simulink model "Task1_SARADC"  (R2026a)
settings: Solver=ode45  StopTime=2000.0000e-009  RelTol=1e-1
values from neighbouring files (symbols this model uses):
  clkper = 10e-9    (= 1e-08)    [Task1_SAR_ADC.m]
  nbit = 8    [Task1_SAR_ADC.m]
undefined symbols (not defined in the file or in its folder): coeff, ramp_slope
libraries: simulink_extras x18, simulink x1
settings Model: Creator=DELL  LastModifiedBy=DELL

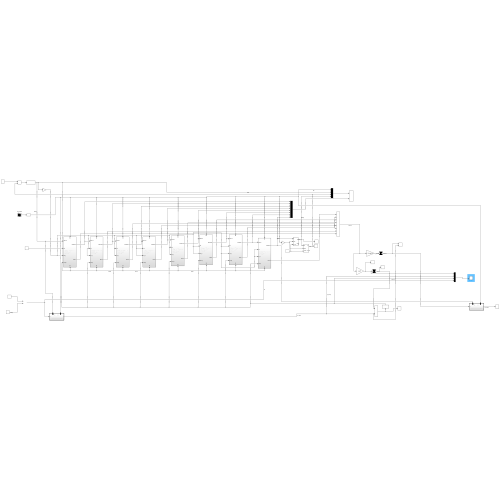
[thumbnail: Simulink's stored preview of the top-level diagram]
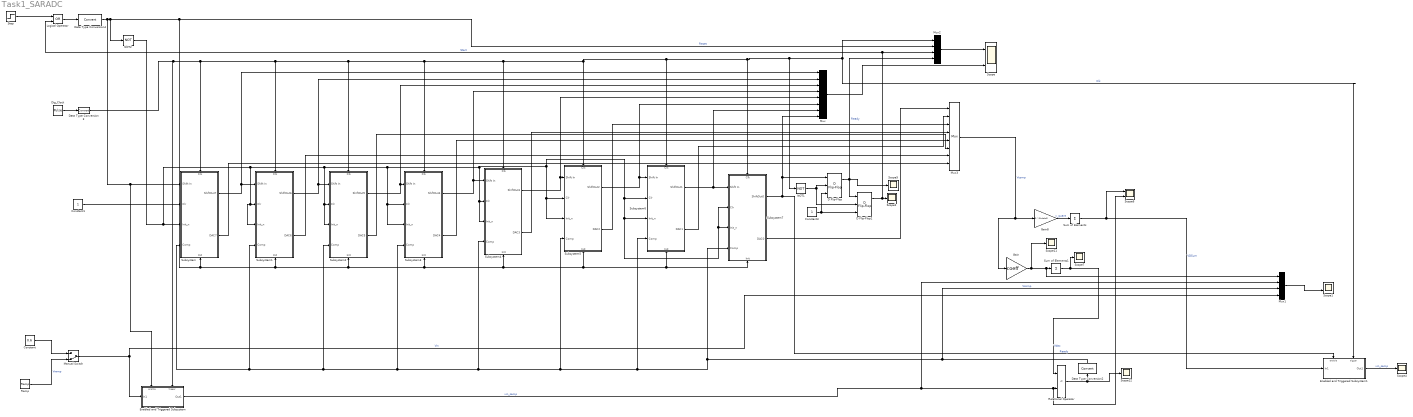
== system Task1_SARADC ==
  Constant : Constant  Value=0.6
  Constant1 : Constant
  Constant3 : Constant
  D Flip-Flop : simulink_extras/Flip Flops/D Flip-Flop
  D Flip-Flop1 : simulink_extras/Flip Flops/D Flip-Flop
  Data Type Conversion2 : DataTypeConversion  SaturateOnIntegerOverflow=off  RndMeth=Floor
  Data Type Conversion3 : DataTypeConversion  SaturateOnIntegerOverflow=off  RndMeth=Floor
  Data Type Conversion4 : DataTypeConversion  SaturateOnIntegerOverflow=off  RndMeth=Floor
  Dig_Clock : DiscretePulseGenerator  PulseType=Time based  Period=clkper  PulseWidth=50  PhaseDelay=clkper/2
  Enabled and Triggered Subsystem : Subsystem  TreatAsAtomicUnit=on
  Enabled and Triggered Subsystem1 : Subsystem  TreatAsAtomicUnit=on
  Gain : Gain  Gain=coeff
  Gain8 : Gain  Gain=2.^(0:nbit-1)
  Logical Operator : Logic  Operator=OR  AllPortsSameDT=off  OutDataTypeStr=boolean
  Manual Switch : ManualSwitch  CurrentSetting=0
  Mux : Mux  Inputs=8
  Mux1 : Mux
  Mux2 : Mux
  Mux3 : Mux  Inputs=8
      settings: DisplayOption=signals
  NOT1 : Logic  Operator=NOT  IconShape=distinctive  AllPortsSameDT=off  OutDataTypeStr=boolean
  NOT2 : Logic  Operator=NOT  IconShape=distinctive  AllPortsSameDT=off  OutDataTypeStr=boolean
  Ramp : simulink/Sources/Ramp  slope=ramp_slope  start=0  InitialOutput=0
  Relational Operator : RelationalOperator  Operator=<  OutDataTypeStr=Inherit: Inherit via back propagation  ZeroCross=off  RndMeth=Simplest  InputSameDT=off
  Scope : Scope  NumInputPorts=2
      settings: ActiveDisplayYMinimum=-0.54674862155056214  ActiveDisplayYMaximum=1.3000706831857676
  Scope1 : Scope  NumInputPorts=2
      settings: ActiveDisplayYMinimum=-0.12499999999999997  ActiveDisplayYMaximum=1.125
  Scope{2,4..5,7,11..12} (6 alike) : Scope
      Scope11 settings: ActiveDisplayYMinimum=-0.1758076641338111  ActiveDisplayYMaximum=0.62186831242868923  DataLoggingVariableName=ScopeData11
      Scope12 settings: ActiveDisplayYMinimum=-0.36561657895351263  ActiveDisplayYMaximum=2.6050694753501595  DataLoggingVariableName=ScopeData12
      Scope2 settings: ActiveDisplayYMinimum=-1.3330651620292413  ActiveDisplayYMaximum=1.0979473379707596  DataLoggingVariableName=ScopeData2
      Scope4 settings: ActiveDisplayYMinimum=-19.124999999999996  ActiveDisplayYMaximum=172.125  DataLoggingVariableName=ScopeData4
      Scope5 settings: ActiveDisplayYMinimum=-1.3892683507462689  ActiveDisplayYMaximum=1.1632947742537318  DataLoggingVariableName=ScopeData5
      Scope7 settings: ActiveDisplayYMinimum=0.44799066402998711  ActiveDisplayYMaximum=0.80442430415689781  DataLoggingVariableName=ScopeData7
  Scope6 : Scope  NumInputPorts=2
      settings: ActiveDisplayYMinimum=-0.10120646692995705  ActiveDisplayYMaximum=1.442692848005839  DataLoggingVariableName=ScopeData6
  Step : Step  Time=clkper  InitialValue=1  FinalValue=0  SampleTime=0
  Subsystem : Subsystem
      settings: PortSchema="{\"entries\":[{\"content\":{\"sides\":[{\"content\":{\"connectorIds\":[\"In1\",\"In2\",\"In3\",\"In4\"]},\"type\":\"ConnectorPlacement.EquallySpacedRectSide\",\"uuid\":\"4452d4c9-2c94-4eae-a6e2-4cf382435c99\"},{\"content\":{\"connectorIds\":[\"Out1\",\"Out2\"],\"side\":\"RIGHT\"},\"type\":\"ConnectorPlacement.EquallySpacedRectSide\",\"uuid\":\"79b24006-096d-4e7e-bd78-a09668d939f4\"},{\"content\":{\"connectorIds\":[\"In5\"],\"side\":\"TOP\"},\"type\":\"ConnectorPlacement.EquallySpacedRectSide\",\"uuid\":\"70478980-d173-4313-b429-e16315b93c93\"},{\"content\":{\"connectorIds\":[\"In6\"],\"side\":\"BOTTOM\"},\"type\":\"ConnectorPlacement.EquallySpacedRectSide\",\"uuid\":\"51cf5911-55bd-40df-b60a-63c48afaa832\"}]},\"type\":\"ConnectorPlacement.EquallySpacedConnector\",\"uuid\":\"6f1f0179-5d91-4253-8aff-d4c324a5668e\"}],\"packageUris\":[\"http://schema.mathworks.com/mf0/Connector/R2020b\"],\"version\":\"1.0\"}"
  Subsystem1 : Subsystem
      settings: PortSchema="{\"entries\":[{\"content\":{\"sides\":[{\"content\":{\"connectorIds\":[\"In1\",\"In2\",\"In3\",\"In4\"]},\"type\":\"ConnectorPlacement.EquallySpacedRectSide\",\"uuid\":\"4452d4c9-2c94-4eae-a6e2-4cf382435c99\"},{\"content\":{\"connectorIds\":[\"Out1\",\"Out2\"],\"side\":\"RIGHT\"},\"type\":\"ConnectorPlacement.EquallySpacedRectSide\",\"uuid\":\"79b24006-096d-4e7e-bd78-a09668d939f4\"},{\"content\":{\"connectorIds\":[\"In5\"],\"side\":\"TOP\"},\"type\":\"ConnectorPlacement.EquallySpacedRectSide\",\"uuid\":\"70478980-d173-4313-b429-e16315b93c93\"},{\"content\":{\"connectorIds\":[\"In6\"],\"side\":\"BOTTOM\"},\"type\":\"ConnectorPlacement.EquallySpacedRectSide\",\"uuid\":\"51cf5911-55bd-40df-b60a-63c48afaa832\"}]},\"type\":\"ConnectorPlacement.EquallySpacedConnector\",\"uuid\":\"6f1f0179-5d91-4253-8aff-d4c324a5668e\"}],\"packageUris\":[\"http://schema.mathworks.com/mf0/Connector/R2020b\"],\"version\":\"1.0\"}"
  Subsystem2 : Subsystem
      settings: PortSchema="{\"entries\":[{\"content\":{\"sides\":[{\"content\":{\"connectorIds\":[\"In1\",\"In2\",\"In3\",\"In4\"]},\"type\":\"ConnectorPlacement.EquallySpacedRectSide\",\"uuid\":\"4452d4c9-2c94-4eae-a6e2-4cf382435c99\"},{\"content\":{\"connectorIds\":[\"Out1\",\"Out2\"],\"side\":\"RIGHT\"},\"type\":\"ConnectorPlacement.EquallySpacedRectSide\",\"uuid\":\"79b24006-096d-4e7e-bd78-a09668d939f4\"},{\"content\":{\"connectorIds\":[\"In5\"],\"side\":\"TOP\"},\"type\":\"ConnectorPlacement.EquallySpacedRectSide\",\"uuid\":\"70478980-d173-4313-b429-e16315b93c93\"},{\"content\":{\"connectorIds\":[\"In6\"],\"side\":\"BOTTOM\"},\"type\":\"ConnectorPlacement.EquallySpacedRectSide\",\"uuid\":\"51cf5911-55bd-40df-b60a-63c48afaa832\"}]},\"type\":\"ConnectorPlacement.EquallySpacedConnector\",\"uuid\":\"6f1f0179-5d91-4253-8aff-d4c324a5668e\"}],\"packageUris\":[\"http://schema.mathworks.com/mf0/Connector/R2020b\"],\"version\":\"1.0\"}"
  Subsystem3 : Subsystem
      settings: PortSchema="{\"entries\":[{\"content\":{\"sides\":[{\"content\":{\"connectorIds\":[\"In1\",\"In2\",\"In3\",\"In4\"]},\"type\":\"ConnectorPlacement.EquallySpacedRectSide\",\"uuid\":\"4452d4c9-2c94-4eae-a6e2-4cf382435c99\"},{\"content\":{\"connectorIds\":[\"Out1\",\"Out2\"],\"side\":\"RIGHT\"},\"type\":\"ConnectorPlacement.EquallySpacedRectSide\",\"uuid\":\"79b24006-096d-4e7e-bd78-a09668d939f4\"},{\"content\":{\"connectorIds\":[\"In5\"],\"side\":\"TOP\"},\"type\":\"ConnectorPlacement.EquallySpacedRectSide\",\"uuid\":\"70478980-d173-4313-b429-e16315b93c93\"},{\"content\":{\"connectorIds\":[\"In6\"],\"side\":\"BOTTOM\"},\"type\":\"ConnectorPlacement.EquallySpacedRectSide\",\"uuid\":\"51cf5911-55bd-40df-b60a-63c48afaa832\"}]},\"type\":\"ConnectorPlacement.EquallySpacedConnector\",\"uuid\":\"6f1f0179-5d91-4253-8aff-d4c324a5668e\"}],\"packageUris\":[\"http://schema.mathworks.com/mf0/Connector/R2020b\"],\"version\":\"1.0\"}"
  Subsystem4 : Subsystem
      settings: PortSchema="{\"entries\":[{\"content\":{\"sides\":[{\"content\":{\"connectorIds\":[\"In1\",\"In2\",\"In3\",\"In4\"]},\"type\":\"ConnectorPlacement.EquallySpacedRectSide\",\"uuid\":\"4452d4c9-2c94-4eae-a6e2-4cf382435c99\"},{\"content\":{\"connectorIds\":[\"Out1\",\"Out2\"],\"side\":\"RIGHT\"},\"type\":\"ConnectorPlacement.EquallySpacedRectSide\",\"uuid\":\"79b24006-096d-4e7e-bd78-a09668d939f4\"},{\"content\":{\"connectorIds\":[\"In5\"],\"side\":\"TOP\"},\"type\":\"ConnectorPlacement.EquallySpacedRectSide\",\"uuid\":\"70478980-d173-4313-b429-e16315b93c93\"},{\"content\":{\"connectorIds\":[\"In6\"],\"side\":\"BOTTOM\"},\"type\":\"ConnectorPlacement.EquallySpacedRectSide\",\"uuid\":\"51cf5911-55bd-40df-b60a-63c48afaa832\"}]},\"type\":\"ConnectorPlacement.EquallySpacedConnector\",\"uuid\":\"6f1f0179-5d91-4253-8aff-d4c324a5668e\"}],\"packageUris\":[\"http://schema.mathworks.com/mf0/Connector/R2020b\"],\"version\":\"1.0\"}"
  Subsystem5 : Subsystem
      settings: PortSchema="{\"entries\":[{\"content\":{\"sides\":[{\"content\":{\"connectorIds\":[\"In1\",\"In2\",\"In3\",\"In4\"]},\"type\":\"ConnectorPlacement.EquallySpacedRectSide\",\"uuid\":\"4452d4c9-2c94-4eae-a6e2-4cf382435c99\"},{\"content\":{\"connectorIds\":[\"Out1\",\"Out2\"],\"side\":\"RIGHT\"},\"type\":\"ConnectorPlacement.EquallySpacedRectSide\",\"uuid\":\"79b24006-096d-4e7e-bd78-a09668d939f4\"},{\"content\":{\"connectorIds\":[\"In5\"],\"side\":\"TOP\"},\"type\":\"ConnectorPlacement.EquallySpacedRectSide\",\"uuid\":\"70478980-d173-4313-b429-e16315b93c93\"},{\"content\":{\"connectorIds\":[\"In6\"],\"side\":\"BOTTOM\"},\"type\":\"ConnectorPlacement.EquallySpacedRectSide\",\"uuid\":\"51cf5911-55bd-40df-b60a-63c48afaa832\"}]},\"type\":\"ConnectorPlacement.EquallySpacedConnector\",\"uuid\":\"6f1f0179-5d91-4253-8aff-d4c324a5668e\"}],\"packageUris\":[\"http://schema.mathworks.com/mf0/Connector/R2020b\"],\"version\":\"1.0\"}"
  Subsystem6 : Subsystem
      settings: PortSchema="{\"entries\":[{\"content\":{\"sides\":[{\"content\":{\"connectorIds\":[\"In1\",\"In2\",\"In3\",\"In4\"]},\"type\":\"ConnectorPlacement.EquallySpacedRectSide\",\"uuid\":\"4452d4c9-2c94-4eae-a6e2-4cf382435c99\"},{\"content\":{\"connectorIds\":[\"Out1\",\"Out2\"],\"side\":\"RIGHT\"},\"type\":\"ConnectorPlacement.EquallySpacedRectSide\",\"uuid\":\"79b24006-096d-4e7e-bd78-a09668d939f4\"},{\"content\":{\"connectorIds\":[\"In5\"],\"side\":\"TOP\"},\"type\":\"ConnectorPlacement.EquallySpacedRectSide\",\"uuid\":\"70478980-d173-4313-b429-e16315b93c93\"},{\"content\":{\"connectorIds\":[\"In6\"],\"side\":\"BOTTOM\"},\"type\":\"ConnectorPlacement.EquallySpacedRectSide\",\"uuid\":\"51cf5911-55bd-40df-b60a-63c48afaa832\"}]},\"type\":\"ConnectorPlacement.EquallySpacedConnector\",\"uuid\":\"6f1f0179-5d91-4253-8aff-d4c324a5668e\"}],\"packageUris\":[\"http://schema.mathworks.com/mf0/Connector/R2020b\"],\"version\":\"1.0\"}"
  Subsystem7 : Subsystem
      settings: PortSchema="{\"entries\":[{\"content\":{\"sides\":[{\"content\":{\"connectorIds\":[\"In1\",\"In2\",\"In3\",\"In4\"]},\"type\":\"ConnectorPlacement.EquallySpacedRectSide\",\"uuid\":\"4452d4c9-2c94-4eae-a6e2-4cf382435c99\"},{\"content\":{\"connectorIds\":[\"Out1\",\"Out2\"],\"side\":\"RIGHT\"},\"type\":\"ConnectorPlacement.EquallySpacedRectSide\",\"uuid\":\"79b24006-096d-4e7e-bd78-a09668d939f4\"},{\"content\":{\"connectorIds\":[\"In5\"],\"side\":\"TOP\"},\"type\":\"ConnectorPlacement.EquallySpacedRectSide\",\"uuid\":\"70478980-d173-4313-b429-e16315b93c93\"},{\"content\":{\"connectorIds\":[\"In6\"],\"side\":\"BOTTOM\"},\"type\":\"ConnectorPlacement.EquallySpacedRectSide\",\"uuid\":\"51cf5911-55bd-40df-b60a-63c48afaa832\"}]},\"type\":\"ConnectorPlacement.EquallySpacedConnector\",\"uuid\":\"6f1f0179-5d91-4253-8aff-d4c324a5668e\"}],\"packageUris\":[\"http://schema.mathworks.com/mf0/Connector/R2020b\"],\"version\":\"1.0\"}"
  Sum of Elements : Sum  Inputs=+
  Sum of Elements1 : Sum  Inputs=+
  wires:
  Dig_Clock/1 -> Data Type Conversion3/1
  Data Type Conversion3/1 -> Enabled and Triggered Subsystem/Trigger, Subsystem/5(Clk), Subsystem2/5(Clk), Subsystem3/5(Clk), Subsystem4/5(Clk), Subsystem5/5(Clk), Subsystem6/5(Clk), Enabled and Triggered Subsystem1/Trigger, Mux2/1, NOT1/1, Subsystem7/5(Clk), Subsystem1/5(Clk)  "Clk"
  Subsystem/1(ShiftOut7) -> Mux/1, Subsystem1/1(Shift In)
  Subsystem1/1(ShiftOut6) -> Mux/2, Subsystem2/1(Shift In)
  Subsystem2/1(ShiftOut5) -> Mux/3, Subsystem3/1(Shift In)
  Subsystem3/1(ShiftOut4) -> Mux/4, Subsystem4/1(Shift In)
  Subsystem4/1(ShiftOut3) -> Mux/5, Subsystem5/1(Shift In)
  Subsystem5/1(ShiftOut2) -> Mux/6, Subsystem6/1(Shift In)
  Subsystem6/1(ShiftOut1) -> Mux/7, Subsystem7/1(Shift In)
  Subsystem7/1(ShiftOut0) -> Enabled and Triggered Subsystem1/Enable, D Flip-Flop/1, Mux/8  "Ready"
  Manual Switch/1 -> Enabled and Triggered Subsystem/1(In1), Mux1/4  "Vin"
  Enabled and Triggered Subsystem/1(Out1) -> Mux1/2, Scope6/2, Relational Operator/2  "vin_samp"
  Relational Operator/1 -> Scope12/1, Data Type Conversion2/1
  D Flip-Flop/1 -> Scope5/1, D Flip-Flop1/1, Mux2/4  "Ready"
  Mux/1 -> Scope/2
  Mux2/1 -> Scope/1
  Data Type Conversion2/1 -> Subsystem7/4(Comp), Subsystem6/4(Comp), Subsystem5/4(Comp), Subsystem4/4(Comp), Subsystem3/4(Comp), Subsystem2/4(Comp), Subsystem1/4(Comp), Subsystem/4(Comp), Mux1/3  "Vcomp"
  Enabled and Triggered Subsystem1/1(Out1) -> Scope4/1  "vin_samp"
  Constant1/1 -> Subsystem/2(Clr)
  Gain/1 -> Scope11/1, Mux1/1, Sum of Elements1/1
  Sum of Elements1/1 -> Scope7/1, Relational Operator/1  "Vdac"
  Gain8/1 -> Sum of Elements/1  "v_quant"
  Sum of Elements/1 -> Scope6/1, Enabled and Triggered Subsystem1/1(In1)  "VDSum"
  Constant/1 -> Manual Switch/1
  Ramp/1 -> Manual Switch/2  "Vramp"
  Subsystem7/2(DAC0) -> Mux3/1
  Subsystem6/2(DAC1) -> Mux3/2
  Subsystem5/2(DAC2) -> Mux3/3
  Subsystem4/2(DAC3) -> Mux3/4
  Subsystem3/2(DAC4) -> Mux3/5
  Subsystem2/2(DAC5) -> Mux3/6
  Subsystem1/2(DAC6) -> Mux3/7
  Subsystem/2(DAC7) -> Mux3/8
  Mux3/1 -> Gain/1, Gain8/1  "Vcomp"
  D Flip-Flop1/1 -> Logical Operator/2, Mux2/3, Scope2/1  "Start"
  NOT1/1 -> D Flip-Flop/2, D Flip-Flop1/2
  Constant3/1 -> D Flip-Flop1/3, D Flip-Flop/3
  Step/1 -> Logical Operator/1
  Logical Operator/1 -> Data Type Conversion4/1
  Data Type Conversion4/1 -> Mux2/2, Subsystem/6(Init), Subsystem2/6(Init), Subsystem3/6(Init), Subsystem4/6(Init), Subsystem5/6(Init), Subsystem6/6(Init), Subsystem7/6(Init), Subsystem1/6(Init), NOT2/1, Enabled and Triggered Subsystem/Enable, Subsystem/1(Shift In)  "Reset"
  NOT2/1 -> Subsystem/3(Init_n), Subsystem1/3(Init_n), Subsystem1/2(Clr), Subsystem2/2(Clr), Subsystem2/3(Init_n), Subsystem3/2(Clr), Subsystem3/3(Init_n), Subsystem4/2(Clr), Subsystem4/3(Init_n), Subsystem5/2(Clr), Subsystem5/3(Init_n), Subsystem6/3(Init_n), Subsystem7/2(Clr), Subsystem7/3(Init_n), Subsystem6/2(Clr)
  Mux1/1 -> Scope1/2

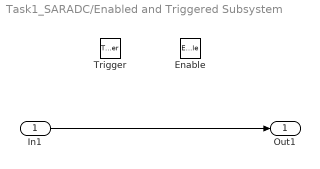
== system Task1_SARADC/Enabled and Triggered Subsystem ==
  In1 : Inport
  Enable : EnablePort
  Trigger : TriggerPort  VariantControl=(inherit)
  Out1 : Outport
  wires:
  In1/1 -> Out1/1

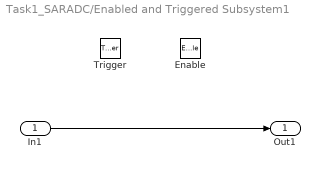
== system Task1_SARADC/Enabled and Triggered Subsystem1 ==
  In1 : Inport
  Enable : EnablePort
  Trigger : TriggerPort  VariantControl=(inherit)
  Out1 : Outport
  wires:
  In1/1 -> Out1/1

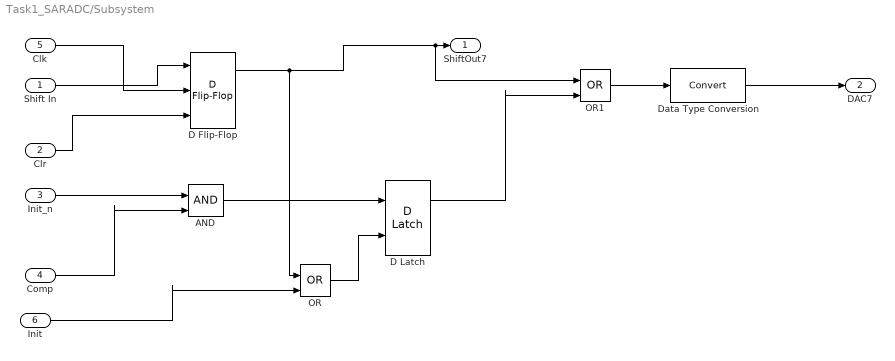
== system Task1_SARADC/Subsystem ==
  Shift In : Inport
  Clr : Inport  Port=2
  Init_n : Inport  Port=3
  Comp : Inport  Port=4
  Clk : Inport  Port=5
  Init : Inport  Port=6
  AND : Logic  IconShape=distinctive  AllPortsSameDT=off  OutDataTypeStr=boolean
  D Flip-Flop : simulink_extras/Flip Flops/D Flip-Flop
  D Latch : simulink_extras/Flip Flops/D Latch
  Data Type Conversion : DataTypeConversion  SaturateOnIntegerOverflow=off  RndMeth=Floor
  OR : Logic  Operator=OR  IconShape=distinctive  AllPortsSameDT=off  OutDataTypeStr=boolean
  OR1 : Logic  Operator=OR  IconShape=distinctive  AllPortsSameDT=off  OutDataTypeStr=boolean
  ShiftOut7 : Outport
  DAC7 : Outport  Port=2
  wires:
  D Flip-Flop/1 -> OR/1, OR1/1, ShiftOut7/1
  Clk/1 -> D Flip-Flop/2
  Shift In/1 -> D Flip-Flop/1
  Clr/1 -> D Flip-Flop/3
  Init_n/1 -> AND/1
  Comp/1 -> AND/2
  AND/1 -> D Latch/1
  Init/1 -> OR/2
  OR/1 -> D Latch/2
  D Latch/1 -> OR1/2
  OR1/1 -> Data Type Conversion/1
  Data Type Conversion/1 -> DAC7/1

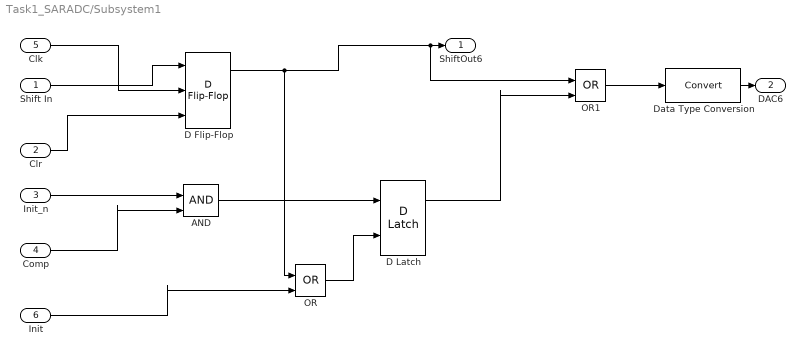
== system Task1_SARADC/Subsystem1 ==
  Shift In : Inport
  Clr : Inport  Port=2
  Init_n : Inport  Port=3
  Comp : Inport  Port=4
  Clk : Inport  Port=5
  Init : Inport  Port=6
  AND : Logic  IconShape=distinctive  AllPortsSameDT=off  OutDataTypeStr=boolean
  D Flip-Flop : simulink_extras/Flip Flops/D Flip-Flop
  D Latch : simulink_extras/Flip Flops/D Latch
  Data Type Conversion : DataTypeConversion  SaturateOnIntegerOverflow=off  RndMeth=Floor
  OR : Logic  Operator=OR  IconShape=distinctive  AllPortsSameDT=off  OutDataTypeStr=boolean
  OR1 : Logic  Operator=OR  IconShape=distinctive  AllPortsSameDT=off  OutDataTypeStr=boolean
  ShiftOut6 : Outport
  DAC6 : Outport  Port=2
  wires:
  D Flip-Flop/1 -> OR/1, OR1/1, ShiftOut6/1
  Clk/1 -> D Flip-Flop/2
  Shift In/1 -> D Flip-Flop/1
  Clr/1 -> D Flip-Flop/3
  Init_n/1 -> AND/1
  Comp/1 -> AND/2
  AND/1 -> D Latch/1
  Init/1 -> OR/2
  OR/1 -> D Latch/2
  D Latch/1 -> OR1/2
  OR1/1 -> Data Type Conversion/1
  Data Type Conversion/1 -> DAC6/1

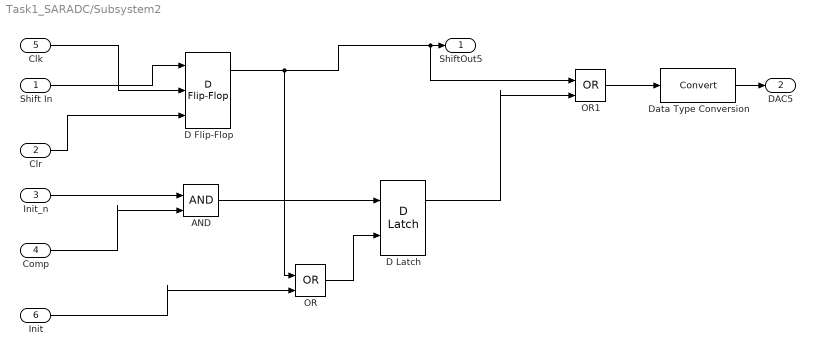
== system Task1_SARADC/Subsystem2 ==
  Shift In : Inport
  Clr : Inport  Port=2
  Init_n : Inport  Port=3
  Comp : Inport  Port=4
  Clk : Inport  Port=5
  Init : Inport  Port=6
  AND : Logic  IconShape=distinctive  AllPortsSameDT=off  OutDataTypeStr=boolean
  D Flip-Flop : simulink_extras/Flip Flops/D Flip-Flop
  D Latch : simulink_extras/Flip Flops/D Latch
  Data Type Conversion : DataTypeConversion  SaturateOnIntegerOverflow=off  RndMeth=Floor
  OR : Logic  Operator=OR  IconShape=distinctive  AllPortsSameDT=off  OutDataTypeStr=boolean
  OR1 : Logic  Operator=OR  IconShape=distinctive  AllPortsSameDT=off  OutDataTypeStr=boolean
  ShiftOut5 : Outport
  DAC5 : Outport  Port=2
  wires:
  D Flip-Flop/1 -> OR/1, OR1/1, ShiftOut5/1
  Clk/1 -> D Flip-Flop/2
  Shift In/1 -> D Flip-Flop/1
  Clr/1 -> D Flip-Flop/3
  Init_n/1 -> AND/1
  Comp/1 -> AND/2
  AND/1 -> D Latch/1
  Init/1 -> OR/2
  OR/1 -> D Latch/2
  D Latch/1 -> OR1/2
  OR1/1 -> Data Type Conversion/1
  Data Type Conversion/1 -> DAC5/1

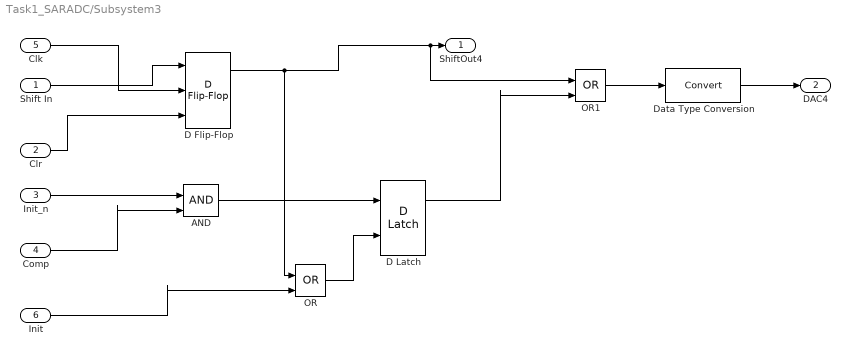
== system Task1_SARADC/Subsystem3 ==
  Shift In : Inport
  Clr : Inport  Port=2
  Init_n : Inport  Port=3
  Comp : Inport  Port=4
  Clk : Inport  Port=5
  Init : Inport  Port=6
  AND : Logic  IconShape=distinctive  AllPortsSameDT=off  OutDataTypeStr=boolean
  D Flip-Flop : simulink_extras/Flip Flops/D Flip-Flop
  D Latch : simulink_extras/Flip Flops/D Latch
  Data Type Conversion : DataTypeConversion  SaturateOnIntegerOverflow=off  RndMeth=Floor
  OR : Logic  Operator=OR  IconShape=distinctive  AllPortsSameDT=off  OutDataTypeStr=boolean
  OR1 : Logic  Operator=OR  IconShape=distinctive  AllPortsSameDT=off  OutDataTypeStr=boolean
  ShiftOut4 : Outport
  DAC4 : Outport  Port=2
  wires:
  D Flip-Flop/1 -> OR/1, OR1/1, ShiftOut4/1
  Clk/1 -> D Flip-Flop/2
  Shift In/1 -> D Flip-Flop/1
  Clr/1 -> D Flip-Flop/3
  Init_n/1 -> AND/1
  Comp/1 -> AND/2
  AND/1 -> D Latch/1
  Init/1 -> OR/2
  OR/1 -> D Latch/2
  D Latch/1 -> OR1/2
  OR1/1 -> Data Type Conversion/1
  Data Type Conversion/1 -> DAC4/1

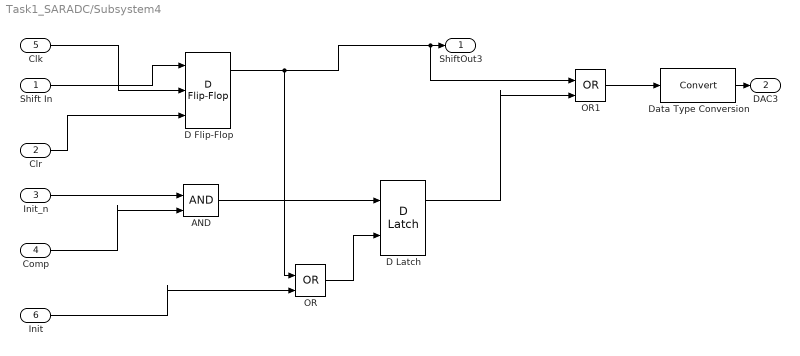
== system Task1_SARADC/Subsystem4 ==
  Shift In : Inport
  Clr : Inport  Port=2
  Init_n : Inport  Port=3
  Comp : Inport  Port=4
  Clk : Inport  Port=5
  Init : Inport  Port=6
  AND : Logic  IconShape=distinctive  AllPortsSameDT=off  OutDataTypeStr=boolean
  D Flip-Flop : simulink_extras/Flip Flops/D Flip-Flop
  D Latch : simulink_extras/Flip Flops/D Latch
  Data Type Conversion : DataTypeConversion  SaturateOnIntegerOverflow=off  RndMeth=Floor
  OR : Logic  Operator=OR  IconShape=distinctive  AllPortsSameDT=off  OutDataTypeStr=boolean
  OR1 : Logic  Operator=OR  IconShape=distinctive  AllPortsSameDT=off  OutDataTypeStr=boolean
  ShiftOut3 : Outport
  DAC3 : Outport  Port=2
  wires:
  D Flip-Flop/1 -> OR/1, OR1/1, ShiftOut3/1
  Clk/1 -> D Flip-Flop/2
  Shift In/1 -> D Flip-Flop/1
  Clr/1 -> D Flip-Flop/3
  Init_n/1 -> AND/1
  Comp/1 -> AND/2
  AND/1 -> D Latch/1
  Init/1 -> OR/2
  OR/1 -> D Latch/2
  D Latch/1 -> OR1/2
  OR1/1 -> Data Type Conversion/1
  Data Type Conversion/1 -> DAC3/1

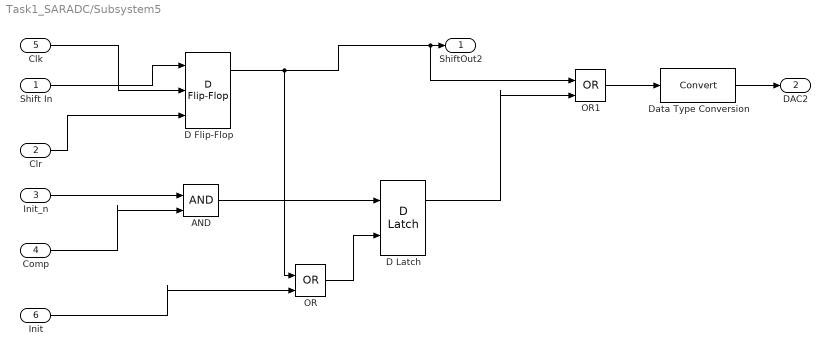
== system Task1_SARADC/Subsystem5 ==
  Shift In : Inport
  Clr : Inport  Port=2
  Init_n : Inport  Port=3
  Comp : Inport  Port=4
  Clk : Inport  Port=5
  Init : Inport  Port=6
  AND : Logic  IconShape=distinctive  AllPortsSameDT=off  OutDataTypeStr=boolean
  D Flip-Flop : simulink_extras/Flip Flops/D Flip-Flop
  D Latch : simulink_extras/Flip Flops/D Latch
  Data Type Conversion : DataTypeConversion  SaturateOnIntegerOverflow=off  RndMeth=Floor
  OR : Logic  Operator=OR  IconShape=distinctive  AllPortsSameDT=off  OutDataTypeStr=boolean
  OR1 : Logic  Operator=OR  IconShape=distinctive  AllPortsSameDT=off  OutDataTypeStr=boolean
  ShiftOut2 : Outport
  DAC2 : Outport  Port=2
  wires:
  D Flip-Flop/1 -> OR/1, OR1/1, ShiftOut2/1
  Clk/1 -> D Flip-Flop/2
  Shift In/1 -> D Flip-Flop/1
  Clr/1 -> D Flip-Flop/3
  Init_n/1 -> AND/1
  Comp/1 -> AND/2
  AND/1 -> D Latch/1
  Init/1 -> OR/2
  OR/1 -> D Latch/2
  D Latch/1 -> OR1/2
  OR1/1 -> Data Type Conversion/1
  Data Type Conversion/1 -> DAC2/1

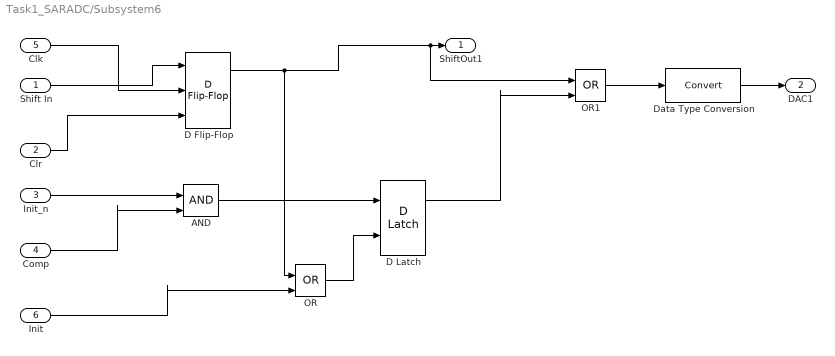
== system Task1_SARADC/Subsystem6 ==
  Shift In : Inport
  Clr : Inport  Port=2
  Init_n : Inport  Port=3
  Comp : Inport  Port=4
  Clk : Inport  Port=5
  Init : Inport  Port=6
  AND : Logic  IconShape=distinctive  AllPortsSameDT=off  OutDataTypeStr=boolean
  D Flip-Flop : simulink_extras/Flip Flops/D Flip-Flop
  D Latch : simulink_extras/Flip Flops/D Latch
  Data Type Conversion : DataTypeConversion  SaturateOnIntegerOverflow=off  RndMeth=Floor
  OR : Logic  Operator=OR  IconShape=distinctive  AllPortsSameDT=off  OutDataTypeStr=boolean
  OR1 : Logic  Operator=OR  IconShape=distinctive  AllPortsSameDT=off  OutDataTypeStr=boolean
  ShiftOut1 : Outport
  DAC1 : Outport  Port=2
  wires:
  D Flip-Flop/1 -> OR/1, OR1/1, ShiftOut1/1
  Clk/1 -> D Flip-Flop/2
  Shift In/1 -> D Flip-Flop/1
  Clr/1 -> D Flip-Flop/3
  Init_n/1 -> AND/1
  Comp/1 -> AND/2
  AND/1 -> D Latch/1
  Init/1 -> OR/2
  OR/1 -> D Latch/2
  D Latch/1 -> OR1/2
  OR1/1 -> Data Type Conversion/1
  Data Type Conversion/1 -> DAC1/1

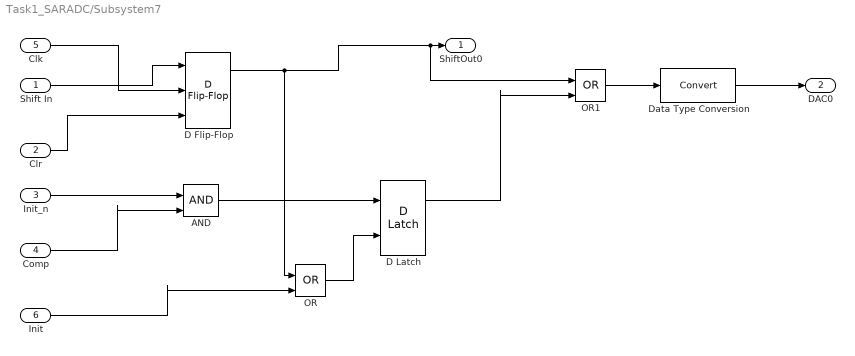
== system Task1_SARADC/Subsystem7 ==
  Shift In : Inport
  Clr : Inport  Port=2
  Init_n : Inport  Port=3
  Comp : Inport  Port=4
  Clk : Inport  Port=5
  Init : Inport  Port=6
  AND : Logic  IconShape=distinctive  AllPortsSameDT=off  OutDataTypeStr=boolean
  D Flip-Flop : simulink_extras/Flip Flops/D Flip-Flop
  D Latch : simulink_extras/Flip Flops/D Latch
  Data Type Conversion : DataTypeConversion  SaturateOnIntegerOverflow=off  RndMeth=Floor
  OR : Logic  Operator=OR  IconShape=distinctive  AllPortsSameDT=off  OutDataTypeStr=boolean
  OR1 : Logic  Operator=OR  IconShape=distinctive  AllPortsSameDT=off  OutDataTypeStr=boolean
  ShiftOut0 : Outport
  DAC0 : Outport  Port=2
  wires:
  D Flip-Flop/1 -> OR/1, OR1/1, ShiftOut0/1
  Clk/1 -> D Flip-Flop/2
  Shift In/1 -> D Flip-Flop/1
  Clr/1 -> D Flip-Flop/3
  Init_n/1 -> AND/1
  Comp/1 -> AND/2
  AND/1 -> D Latch/1
  Init/1 -> OR/2
  OR/1 -> D Latch/2
  D Latch/1 -> OR1/2
  OR1/1 -> Data Type Conversion/1
  Data Type Conversion/1 -> DAC0/1
